simulink model "pmsm_model_Lab4_sensorless_st_R2022a"  (R2022a)
settings: Solver=ode4  StartTime=0.0  StopTime=Tf  FixedStep=Tsim  MaxStep=Tsim  MinStep=Tsim/100  RelTol=1e-3
values from neighbouring files (symbols this model uses):
  b = 0    [pmsm_param_Lab4_2024_st.m]
  C32 = [ 1       0 ... (first row only)    [pmsm_param_Lab1_2025.m]    (also in pmsm_param_Lab2_2025_st.m; pmsm_param_Lab3_st.m; pmsm_param_Lab4_2024_st.m)
  C32inv = 2/3*[1    -1/2        -1/2 ... (first row only)    [pmsm_param_Lab1_2025.m]    (also in pmsm_param_Lab2_2025_st.m; pmsm_param_Lab3_st.m; pmsm_param_Lab4_2024_st.m)
  C33 = C32*C32inv    [pmsm_param_Lab1_2025.m]    (also in pmsm_param_Lab2_2025_st.m; pmsm_param_Lab3_st.m; pmsm_param_Lab4_2024_st.m)
  Cb = 500e-6    (= 0.0005)    [pmsm_param_Lab3_st.m]    (also in pmsm_param_Lab4_2024_st.m)
  dTm0 = 0.20*Tmrated    (= 48)    [pmsm_param_Lab2_2025_st.m]    (also in pmsm_param_Lab3_st.m; pmsm_param_Lab4_2024_st.m = 120)
  Dyno = 1    [pmsm_param_Lab3_st.m]    (also in pmsm_param_Lab4_2024_st.m = 0)
  f = 15e-3    (= 0.015)    [pmsm_param_Lab1_2025.m]    (also in pmsm_param_Lab2_2025_st.m; pmsm_param_Lab3_st.m; pmsm_param_Lab4_2024_st.m)
  frslvr = 1/Ts    (= 10000)    [pmsm_param_Lab4_2024_st.m]
  Id0 = 0    [pmsm_param_Lab1_2025.m]    (also in pmsm_param_Lab2_2025_st.m; pmsm_param_Lab3_st.m = interp1(Tref,Idopt,Tm0); pmsm_param_Lab4_2024_st.m = interp1(Tref,Idopt,Tm0))
  Idc0 = Pe0/VDC    [pmsm_param_Lab3_st.m]    (also in pmsm_param_Lab4_2024_st.m)
  Idopt = zeros(1,NT)    [pmsm_param_Lab3_st.m]    (also in pmsm_param_Lab4_2024_st.m)
  Iq0 = 2/3*Tm0/(Pp*Psif)    (= 0)    [pmsm_param_Lab1_2025.m]    (also in pmsm_param_Lab2_2025_st.m = 119.926066866; pmsm_param_Lab3_st.m = interp1(Tref,Iqopt,Tm0); pmsm_param_Lab4_2024_st.m = interp1(Tref,Iqopt,Tm0))
  Iqopt = zeros(1,NT)    [pmsm_param_Lab3_st.m]    (also in pmsm_param_Lab4_2024_st.m)
  J = 100e-3    (= 0.1)    [pmsm_param_Lab1_2025.m]    (also in pmsm_param_Lab2_2025_st.m; pmsm_param_Lab3_st.m; pmsm_param_Lab4_2024_st.m)
  Kid = Kpd / tid    (= 282.743237724)    [pmsm_param_Lab2_2025_st.m]    (also in pmsm_param_Lab3_st.m = 180; pmsm_param_Lab4_2024_st.m = 180)
  Kiq = Kpq / tiq    (= 282.743237724)    [pmsm_param_Lab2_2025_st.m]    (also in pmsm_param_Lab3_st.m = 180; pmsm_param_Lab4_2024_st.m = 180)
  kL = 0.750    (= 0.75)    [pmsm_param_Lab1_2025.m]    (also in pmsm_param_Lab2_2025_st.m; pmsm_param_Lab3_st.m; pmsm_param_Lab4_2024_st.m)
  Kpd = (3*Ld0) / tr    (= 6.28318306054)    [pmsm_param_Lab2_2025_st.m]    (also in pmsm_param_Lab3_st.m = 3; pmsm_param_Lab4_2024_st.m = 3)
  Kpll = 1    [pmsm_param_Lab4_2024_st.m]
  Kpq = (3 * Lq0) / tr    (= 3.14159153027)    [pmsm_param_Lab2_2025_st.m]    (also in pmsm_param_Lab3_st.m = 6; pmsm_param_Lab4_2024_st.m = 6)
  ksi = 0    [pmsm_param_Lab4_2024_st.m]
  Lb = 20e-6    (= 2e-05)    [pmsm_param_Lab3_st.m]    (also in pmsm_param_Lab4_2024_st.m)
  Ld0 = 2.0*Ld    (= 0.002)    [pmsm_param_Lab2_2025_st.m]    (also in pmsm_param_Lab3_st.m = 0.001; pmsm_param_Lab4_2024_st.m = 0.001)
  Lq0 = 0.5*Lq    (= 0.001)    [pmsm_param_Lab2_2025_st.m]    (also in pmsm_param_Lab3_st.m = 0.002; pmsm_param_Lab4_2024_st.m = 0.002)
  Pe0 = 3/2*(Vd0*Id0+Vq0*Iq0)    [pmsm_param_Lab2_2025_st.m]    (also in pmsm_param_Lab3_st.m; pmsm_param_Lab4_2024_st.m)
  Pp = 4    [pmsm_param_Lab1_2025.m]    (also in pmsm_param_Lab2_2025_st.m; pmsm_param_Lab3_st.m; pmsm_param_Lab4_2024_st.m)
  ppll = cell2mat(ppll)    [pmsm_param_Lab4_2024_st.m]
  Psid0 = interpn(Idv,Iqv,Psidd,Id0,Iq0)    [pmsm_param_Lab1_2025.m]    (also in pmsm_param_Lab2_2025_st.m; pmsm_param_Lab3_st.m; pmsm_param_Lab4_2024_st.m)
  Psif0 = 1.0*Psif    (= 0.167)    [pmsm_param_Lab2_2025_st.m]    (also in pmsm_param_Lab3_st.m; pmsm_param_Lab4_2024_st.m)
  Psiq0 = interpn(Idv,Iqv,Psiqq,Id0,Iq0)    [pmsm_param_Lab1_2025.m]    (also in pmsm_param_Lab2_2025_st.m; pmsm_param_Lab3_st.m; pmsm_param_Lab4_2024_st.m)
  Qbat = 72*3600    (= 259200)    [pmsm_param_Lab3_st.m]    (also in pmsm_param_Lab4_2024_st.m)
  RateTm = 10000    [pmsm_param_Lab3_st.m]    (also in pmsm_param_Lab4_2024_st.m)
  rb = 80e-3    (= 0.08)    [pmsm_param_Lab3_st.m]    (also in pmsm_param_Lab4_2024_st.m)
  Rs = 60e-3    (= 0.06)    [pmsm_param_Lab1_2025.m]    (also in pmsm_param_Lab2_2025_st.m; pmsm_param_Lab3_st.m; pmsm_param_Lab4_2024_st.m)
  Rs0 = 1.5*Rs    (= 0.09)    [pmsm_param_Lab2_2025_st.m]    (also in pmsm_param_Lab3_st.m = 0.06; pmsm_param_Lab4_2024_st.m = 0.06)
  SOC0 = 0.50    (= 0.5)    [pmsm_param_Lab3_st.m]    (also in pmsm_param_Lab4_2024_st.m)
  Thetae0 = 0    [pmsm_param_Lab1_2025.m]    (also in pmsm_param_Lab2_2025_st.m; pmsm_param_Lab3_st.m; pmsm_param_Lab4_2024_st.m)
  Tm0 = (kL+f)*Wm0    (= 0)    [pmsm_param_Lab1_2025.m]    (also in pmsm_param_Lab2_2025_st.m = 120.165919; pmsm_param_Lab3_st.m = 192.2654704; pmsm_param_Lab4_2024_st.m)
  Tp = 100e-6    (= 0.0001)    [pmsm_param_Lab2_2025_st.m]    (also in pmsm_param_Lab3_st.m; pmsm_param_Lab4_2024_st.m)
  Tref = -Tmax:Tmax/100:Tmax    [pmsm_param_Lab3_st.m]    (also in pmsm_param_Lab4_2024_st.m)
  Ts = Tsim    [pmsm_param_Lab2_2025_st.m]    (also in pmsm_param_Lab3_st.m = 0.0001; pmsm_param_Lab4_2024_st.m = 0.0001)
  Tsim = 1e-6    (= 1e-06)    [pmsm_param_Lab1_2025.m]    (also in pmsm_param_Lab2_2025_st.m = min([Tp Ts])/100; pmsm_param_Lab3_st.m = min([Tp Ts])/100; pmsm_param_Lab4_2024_st.m = min([Tp Ts])/100)
  TSS = Tstep+0.050    (= 0.1)    [pmsm_param_Lab3_st.m]    (also in pmsm_param_Lab4_2024_st.m)
  Tstep = 0.10    (= 0.1)    [pmsm_param_Lab2_2025_st.m]    (also in pmsm_param_Lab3_st.m = 0.05; pmsm_param_Lab4_2024_st.m = 0.05)
  Ud0 = Rs*Id0    (= 0)    [pmsm_param_Lab2_2025_st.m]    (also in pmsm_param_Lab3_st.m; pmsm_param_Lab4_2024_st.m)
  Uq0 = Rs*Iq0    (= 7.19556401196)    [pmsm_param_Lab2_2025_st.m]    (also in pmsm_param_Lab3_st.m = 11.5129024191; pmsm_param_Lab4_2024_st.m = Rs*Iq0)
  Vd0 = Rs*Id0-Pp*Psiq0*Wm0    [pmsm_param_Lab1_2025.m]    (also in pmsm_param_Lab2_2025_st.m = Ud0-Pp*Psiq0*Wm0; pmsm_param_Lab3_st.m = Ud0-Pp*Psiq0*Wm0; pmsm_param_Lab4_2024_st.m = Ud0-Pp*Psiq0*Wm0)
  VDC = 800    [pmsm_param_Lab2_2025_st.m]    (also in pmsm_param_Lab3_st.m; pmsm_param_Lab4_2024_st.m)
  VDC0 = 0.8*VDC    (= 640)    [pmsm_param_Lab3_st.m]    (also in pmsm_param_Lab4_2024_st.m)
  Vp = VDC/2    (= 400)    [pmsm_param_Lab2_2025_st.m]    (also in pmsm_param_Lab3_st.m; pmsm_param_Lab4_2024_st.m)
  Vq0 = Rs*Iq0+Pp*Psid0*Wm0    [pmsm_param_Lab1_2025.m]    (also in pmsm_param_Lab2_2025_st.m = Uq0+Pp*Psid0*Wm0; pmsm_param_Lab3_st.m = Uq0+Pp*Psid0*Wm0; pmsm_param_Lab4_2024_st.m = Uq0+Pp*Psid0*Wm0)
  we0 = Pp*Wm0    (= 0)    [pmsm_param_Lab4_2024_st.m]
  Wm0 = 0    [pmsm_param_Lab1_2025.m]    (also in pmsm_param_Lab2_2025_st.m = 157.079632679; pmsm_param_Lab3_st.m = 251.327412287; pmsm_param_Lab4_2024_st.m)
  zpll = cell2mat(zpll)    [pmsm_param_Lab4_2024_st.m]
undefined symbols (not defined in the file or in its folder): DiscIntNeverNeededParam, Idd, Idrop, Iqq, Isw, kpll, Psidv, Psiqv, SwLoss, Vdrop
libraries: simulink x10
(part 2 of 2)

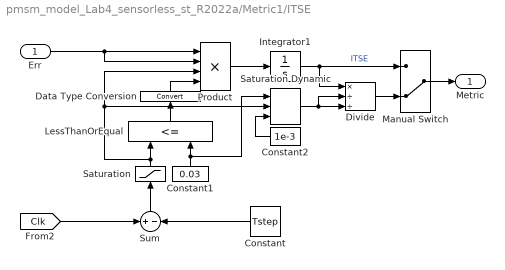
== system pmsm_model_Lab4_sensorless_st_R2022a/Metric1/ITSE ==
  Err : Inport
  Constant : Constant  Value=Tstep
  Constant1 : Constant  Value=0.03
  Constant2 : Constant  Value=1e-3
  Data Type Conversion : DataTypeConversion  SaturateOnIntegerOverflow=off  RndMeth=Floor
  Divide : Product  Inputs=*//
  Integrator1 : Integrator
  LessThanOrEqual : RelationalOperator  Operator=<=  OutDataTypeStr=boolean  RndMeth=Simplest  InputSameDT=off
  Manual Switch : ManualSwitch  CurrentSetting=0
  Product : Product  Inputs=4
  Saturation : Saturate  UpperLimit=inf  LowerLimit=0
  Saturation Dynamic : simulink/Discontinuities/Saturation Dynamic  OutMin=[]  OutMax=[]  OutDataTypeStr=Inherit: Same as second input  OutDataType=fixdt(1, 16)  OutScaling=2^-10  DoSatur=off
  Sum : Sum  Inputs=+|-
  Metric : Outport
  wires:
  Sum/1 -> Saturation/1
  Integrator1/1 -> Divide/1, Manual Switch/1  "ITSE"
  Err/1 -> Product/1, Product/2
  Product/1 -> Integrator1/1
  [Clk] -> Sum/1
  Saturation/1 -> Saturation Dynamic/2, Product/3, LessThanOrEqual/1
  Constant/1 -> Sum/2
  Divide/1 -> Manual Switch/2
  Manual Switch/1 -> Metric/1
  Saturation Dynamic/1 -> Divide/3, Divide/2
  LessThanOrEqual/1 -> Data Type Conversion/1
  Constant1/1 -> Saturation Dynamic/1, LessThanOrEqual/2
  Data Type Conversion/1 -> Product/4
  Constant2/1 -> Saturation Dynamic/3

== system pmsm_model_Lab4_sensorless_st_R2022a/Metric1/LPF ==
  x : Inport
  Gain : Gain  Gain=2*pi*10
  Integrator : Integrator
  Sum : Sum  Inputs=|+-
  xf : Outport
  wires:
  Gain/1 -> Integrator/1
  Sum/1 -> Gain/1
  Integrator/1 -> Sum/2, xf/1
  x/1 -> Sum/1

== system pmsm_model_Lab4_sensorless_st_R2022a/Metric1/RMSE ==
  Err : Inport
  Divide : Product  Inputs=*/
  Integrator1 : Integrator
  Integrator2 : Integrator
  Product : Product  Inputs=3
  Saturation : Saturate  UpperLimit=inf  LowerLimit=1e-3
  Sqrt : Sqrt
  Sqrt1 : Sqrt
  RMSE : Outport
  wires:
  Err/1 -> Product/1, Product/2
  Product/1 -> Integrator1/1
  Integrator1/1 -> Sqrt/1
  Sqrt/1 -> Divide/1
  [SS] -> Product/3, Integrator2/1
  Divide/1 -> RMSE/1
  Integrator2/1 -> Saturation/1
  Saturation/1 -> Sqrt1/1
  Sqrt1/1 -> Divide/2

== system pmsm_model_Lab4_sensorless_st_R2022a/Metric2/LPF ==
  Tm : Inport
  Gain : Gain  Gain=2*pi*10
  Integrator : Integrator  InitialCondition=Tm0
  Sum : Sum  Inputs=|+-
  Tav : Outport
  wires:
  Gain/1 -> Integrator/1
  Integrator/1 -> Tav/1, Sum/2
  Sum/1 -> Gain/1
  Tm/1 -> Sum/1

== system pmsm_model_Lab4_sensorless_st_R2022a/Metric2/Window ==
  "Tav " : Inport
  Dead Zone : DeadZone  LowerValue=-inf  UpperValue=Tstep
  Manual Switch : ManualSwitch
  Product : Product
  Tav : Outport
  wires:
  [SS] -> Manual Switch/1
  Dead Zone/1 -> Manual Switch/2  "ITSE"
  Manual Switch/1 -> Product/2
  Product/1 -> Tav/1
  [Clk] -> Dead Zone/1
  "Tav "/1 -> Product/1

== system pmsm_model_Lab4_sensorless_st_R2022a/Metric3/LPF ==
  Tm : Inport
  Gain : Gain  Gain=2*pi*30
  Integrator : Integrator  InitialCondition=Tm0
  Sum : Sum  Inputs=|+-
  Sum1 : Sum  Inputs=+-|
  Tmh : Outport
  Tm0 : Outport  Port=2
  wires:
  Tm/1 -> Sum1/1, Sum/1
  Integrator/1 -> Sum1/2, Tm0/1, Sum/2
  Sum/1 -> Gain/1
  Sum1/1 -> Tmh/1
  Gain/1 -> Integrator/1

== system pmsm_model_Lab4_sensorless_st_R2022a/Metric3/LPF2 ==
  x : Inport
  Gain : Gain  Gain=2*pi*10
  Integrator : Integrator
  Sum : Sum  Inputs=|+-
  xf : Outport
  wires:
  Gain/1 -> Integrator/1
  Sum/1 -> Gain/1
  Integrator/1 -> Sum/2, xf/1
  x/1 -> Sum/1

== system pmsm_model_Lab4_sensorless_st_R2022a/Metric3/Ripple ==
  Tmh : Inport
  Tm0 : Inport  Port=2
  Divide : Product  Inputs=*//
  Gain : Gain  Gain=100
  Integrator1 : Integrator
  Integrator2 : Integrator
  Product : Product  Inputs=3
  Saturation : Saturate  UpperLimit=inf  LowerLimit=1e-3
  Saturation1 : Saturate  UpperLimit=inf  LowerLimit=1e-3
  Sqrt : Sqrt
  Sqrt1 : Sqrt
  Ripple : Outport
  wires:
  Product/1 -> Integrator1/1
  Integrator1/1 -> Sqrt/1
  Sqrt/1 -> Divide/1
  [SS] -> Integrator2/1, Product/3
  Divide/1 -> Gain/1
  Gain/1 -> Ripple/1
  Integrator2/1 -> Saturation/1
  Saturation/1 -> Sqrt1/1
  Tm0/1 -> Saturation1/1
  Saturation1/1 -> Divide/3
  Sqrt1/1 -> Divide/2
  Tmh/1 -> Product/1, Product/2

== system pmsm_model_Lab4_sensorless_st_R2022a/PMSM/Flux_Current ==
  Psid : Inport
  Psiq : Inport  Port=2
  Id : Lookup_n-D  BreakpointsForDimension1=Psidv  BreakpointsForDimension2=Psiqv  Table=Idd  InternalRulePriority=Speed  RndMeth=Simplest
      settings: InputPortMap=u0,u1
  Iq : Lookup_n-D  BreakpointsForDimension1=Psidv  BreakpointsForDimension2=Psiqv  Table=Iqq  InternalRulePriority=Speed  RndMeth=Simplest
      settings: InputPortMap=u0,u1
  id : Outport
  iq : Outport  Port=2
  wires:
  Psiq/1 -> Iq/2, Id/2
  Psid/1 -> Iq/1, Id/1
  Iq/1 -> iq/1
  Id/1 -> id/1

== system pmsm_model_Lab4_sensorless_st_R2022a/PMSM/abc_dq ==
  abc : Inport
  sin_cos : Inport  Port=2
  Demux : Demux  Outputs=2
      settings: DisplayOption=none
  Demux1 : Demux  Outputs=2
      settings: DisplayOption=none
  Gain3 : Gain  Gain=C32inv  Multiplication=Matrix(K*u)  OutDataTypeStr=Inherit: Same as input  ParamDataTypeStr=Inherit: Same as input
  Mux : Mux  Inputs=2
  Product{,1..3} (4 alike) : Product  InputSameDT=on  RndMeth=Zero  SaturateOnIntegerOverflow=on  OutDataTypeStr=Inherit: Same as first input
  Sum : Sum  Inputs=|++  InputSameDT=on  SaturateOnIntegerOverflow=on  OutDataTypeStr=Inherit: Same as first input
  Sum1 : Sum  Inputs=|-+  InputSameDT=on  SaturateOnIntegerOverflow=on  OutDataTypeStr=Inherit: Same as first input
  dq : Outport
  wires:
  Sum1/1 -> Mux/2
  Mux/1 -> dq/1
  Demux1/1 -> Product2/2, Product1/2
  sin_cos/1 -> Demux1/1
  Demux/2 -> Product3/2, Product1/1
  Gain3/1 -> Demux/1  "alpha_beta"
  abc/1 -> Gain3/1
  Demux1/2 -> Product3/1, Product/2
  Demux/1 -> Product2/1, Product/1
  Sum/1 -> Mux/1
  Product3/1 -> Sum1/2
  Product2/1 -> Sum1/1
  Product1/1 -> Sum/2
  Product/1 -> Sum/1

== system pmsm_model_Lab4_sensorless_st_R2022a/PMSM/dq_abc ==
  dq : Inport
  sin_cos : Inport  Port=2
  Demux1 : Demux  Outputs=2
      settings: DisplayOption=none
  Demux2 : Demux  Outputs=2
      settings: DisplayOption=none
  Gain1 : Gain  Gain=C32  Multiplication=Matrix(K*u)  OutDataTypeStr=Inherit: Same as input  ParamDataTypeStr=Inherit: Same as input
  Mux : Mux  Inputs=2
  Product{,1..3} (4 alike) : Product  InputSameDT=on  RndMeth=Zero  SaturateOnIntegerOverflow=on  OutDataTypeStr=Inherit: Same as first input
  Sum : Sum  Inputs=|+-  InputSameDT=on  SaturateOnIntegerOverflow=on  OutDataTypeStr=Inherit: Same as first input
  Sum1 : Sum  Inputs=|++  InputSameDT=on  SaturateOnIntegerOverflow=on  OutDataTypeStr=Inherit: Same as first input
  abc : Outport
  wires:
  Mux/1 -> Gain1/1
  Demux1/1 -> Product2/2, Product1/2
  sin_cos/1 -> Demux1/1
  dq/1 -> Demux2/1
  Demux1/2 -> Product3/1, Product/2
  Product3/1 -> Sum1/2
  Product2/1 -> Sum1/1
  Product1/1 -> Sum/2
  Product/1 -> Sum/1
  Demux2/1 -> Product/1, Product2/1
  Demux2/2 -> Product3/2, Product1/1
  Sum/1 -> Mux/1
  Sum1/1 -> Mux/2
  Gain1/1 -> abc/1

== system pmsm_model_Lab4_sensorless_st_R2022a/PMSM/sin_cos ==
  thetae : Inport
  Mux1 : Mux  Inputs=2
  Trigonometric Function : Trigonometry
  Trigonometric Function1 : Trigonometry  Operator=cos
  sin_cos : Outport
  wires:
  Trigonometric Function/1 -> Mux1/1
  Trigonometric Function1/1 -> Mux1/2
  thetae/1 -> Trigonometric Function1/1, Trigonometric Function/1
  Mux1/1 -> sin_cos/1

== system pmsm_model_Lab4_sensorless_st_R2022a/Resolver/PLLPositionError ==
  u1 : Inport
  u2 : Inport  Port=2
  Constant : Constant  Value=2*pi
  Gain : Gain  Gain=0.5
  Sum : Sum  Inputs=+-+
  Sum1 : Sum  Inputs=-+|
  teta : Math  Operator=mod  SignedPower=on
  err : Outport
  wires:
  u2/1 -> Sum/2
  Sum/1 -> teta/1
  teta/1 -> Sum1/2
  Constant/1 -> Gain/1, teta/2
  Sum1/1 -> err/1
  u1/1 -> Sum/1
  Gain/1 -> Sum/3, Sum1/1

== system pmsm_model_Lab4_sensorless_st_R2022a/Resolver/PositionEstimationError ==
  u1 : Inport
  u2 : Inport  Port=2
  Constant : Constant  Value=2*pi
  Gain : Gain  Gain=0.5
  Sum : Sum  Inputs=+-+
  Sum1 : Sum  Inputs=-+|
  teta : Math  Operator=mod  SignedPower=on
  err : Outport
  wires:
  Gain/1 -> Sum1/1, Sum/3
  u1/1 -> Sum/1
  Sum1/1 -> err/1
  Constant/1 -> teta/2, Gain/1
  teta/1 -> Sum1/2
  Sum/1 -> teta/1
  u2/1 -> Sum/2

== system pmsm_model_Lab4_sensorless_st_R2022a/Resolver/SimplifiedResolver ==
  Thetae : Inport
  Supply : Inport  Port=2
  Product : Product
  Product1 : Product
  Sum : Sum  Inputs=++|
  Trigonometric Function : Trigonometry  Operator=cos
  Trigonometric Function1 : Trigonometry
  unbalalanced_gain : Gain
  unbalanced_offset : Constant  Value=0
  cosm : Outport
  sinm : Outport  Port=2
  wires:
  unbalalanced_gain/1 -> Sum/2
  Thetae/1 -> Trigonometric Function1/1, Trigonometric Function/1
  Trigonometric Function/1 -> unbalalanced_gain/1
  unbalanced_offset/1 -> Sum/1
  Trigonometric Function1/1 -> Product1/1
  Sum/1 -> Product/1
  Product/1 -> cosm/1
  Product1/1 -> sinm/1
  Supply/1 -> Product/2, Product1/2

== system pmsm_model_Lab4_sensorless_st_R2022a/SPWM/S1 ==
  "C " : Inport
  NOT : Logic  Operator=NOT  IconShape=distinctive  AllPortsSameDT=off  OutDataTypeStr=boolean
  C : Outport
  C* : Outport  Port=2
  wires:
  "C "/1 -> C/1, NOT/1
  NOT/1 -> C*/1

== system pmsm_model_Lab4_sensorless_st_R2022a/SPWM/S2 ==
  "C " : Inport
  NOT : Logic  Operator=NOT  IconShape=distinctive  AllPortsSameDT=off  OutDataTypeStr=boolean
  C : Outport
  C* : Outport  Port=2
  wires:
  NOT/1 -> C*/1
  "C "/1 -> NOT/1, C/1

== system pmsm_model_Lab4_sensorless_st_R2022a/SPWM/S3 ==
  "C " : Inport
  NOT : Logic  Operator=NOT  IconShape=distinctive  AllPortsSameDT=off  OutDataTypeStr=boolean
  C : Outport
  C* : Outport  Port=2
  wires:
  "C "/1 -> C/1, NOT/1
  NOT/1 -> C*/1

== system pmsm_model_Lab4_sensorless_st_R2022a/SPWM/carrier ==
  t : Inport
  Abs : Abs
  Constant2 : Constant  Value=-Vp
  Signal Generator : SignalGenerator  WaveForm=sawtooth  TimeSource=Use external signal  Amplitude=2*Vp  Frequency=1/Tp
  Sum2 : Sum  SaturateOnIntegerOverflow=on
  Vp : Outport
  wires:
  Sum2/1 -> Vp/1
  Constant2/1 -> Sum2/1
  Abs/1 -> Sum2/2
  Signal Generator/1 -> Abs/1
  t/1 -> Signal Generator/1

== system pmsm_model_Lab4_sensorless_st_R2022a/VSI/V1 ==
  C : Inport
  C* : Inport  Port=2
  I : Inport  Port=3
  Vs : Inport  Port=4
  Compare To Zero : simulink/Logic and Bit Operations/Compare To Zero  relop=>  OutDataTypeStr=boolean  ZeroCross=off
  Demux : Demux  Outputs=2
  Leg : CombinatorialLogic  TruthTable=[1 1;0 0;1 1;0.5 1;0 0;0 0;1 1;0.5 1]
  Mux : Mux  Inputs=3
  Product1 : Product  SaturateOnIntegerOverflow=on  OutDataTypeStr=Inherit: Same as first input
  Product3 : Product  SaturateOnIntegerOverflow=on  OutDataTypeStr=Inherit: Same as first input
  Sum1 : Sum  Inputs=-+|  SaturateOnIntegerOverflow=on
  Vdrop : Lookup_n-D  NumberOfTableDimensions=1  BreakpointsForDimension1=Idrop  Table=Vdrop  InternalRulePriority=Speed  RndMeth=Simplest
  V : Outport
  il : Outport  Port=2
  wires:
  Mux/1 -> Leg/1
  I/1 -> Product3/2, Vdrop/1, Compare To Zero/1
  C*/1 -> Mux/3
  C/1 -> Mux/2
  Compare To Zero/1 -> Mux/1
  Leg/1 -> Demux/1
  Demux/1 -> Product1/2
  Vs/1 -> Product1/1
  Sum1/1 -> V/1
  Product3/1 -> il/1
  Demux/2 -> Product3/1
  Product1/1 -> Sum1/2
  Vdrop/1 -> Sum1/1

== system pmsm_model_Lab4_sensorless_st_R2022a/VSI/V2 ==
  C : Inport
  C* : Inport  Port=2
  I : Inport  Port=3
  Vs : Inport  Port=4
  Compare To Zero : simulink/Logic and Bit Operations/Compare To Zero  relop=>  OutDataTypeStr=boolean  ZeroCross=off
  Demux : Demux  Outputs=2
  Leg : CombinatorialLogic  TruthTable=[1 1;0 0;1 1;0.5 1;0 0;0 0;1 1;0.5 1]
  Mux : Mux  Inputs=3
  Product1 : Product  SaturateOnIntegerOverflow=on  OutDataTypeStr=Inherit: Same as first input
  Product3 : Product  SaturateOnIntegerOverflow=on  OutDataTypeStr=Inherit: Same as first input
  Sum1 : Sum  Inputs=-+|  SaturateOnIntegerOverflow=on
  Vdrop : Lookup_n-D  NumberOfTableDimensions=1  BreakpointsForDimension1=Idrop  Table=Vdrop  InternalRulePriority=Speed  RndMeth=Simplest
  V : Outport
  il : Outport  Port=2
  wires:
  Vdrop/1 -> Sum1/1
  Product1/1 -> Sum1/2
  Demux/2 -> Product3/1
  Product3/1 -> il/1
  Sum1/1 -> V/1
  Vs/1 -> Product1/1
  Demux/1 -> Product1/2
  Leg/1 -> Demux/1
  Compare To Zero/1 -> Mux/1
  C/1 -> Mux/2
  C*/1 -> Mux/3
  I/1 -> Compare To Zero/1, Vdrop/1, Product3/2
  Mux/1 -> Leg/1

== system pmsm_model_Lab4_sensorless_st_R2022a/VSI/V3 ==
  C : Inport
  C* : Inport  Port=2
  I : Inport  Port=3
  Vs : Inport  Port=4
  Compare To Zero : simulink/Logic and Bit Operations/Compare To Zero  relop=>  OutDataTypeStr=boolean  ZeroCross=off
  Demux : Demux  Outputs=2
  Leg : CombinatorialLogic  TruthTable=[1 1;0 0;1 1;0.5 1;0 0;0 0;1 1;0.5 1]
  Mux : Mux  Inputs=3
  Product1 : Product  SaturateOnIntegerOverflow=on  OutDataTypeStr=Inherit: Same as first input
  Product3 : Product  SaturateOnIntegerOverflow=on  OutDataTypeStr=Inherit: Same as first input
  Sum1 : Sum  Inputs=-+|  SaturateOnIntegerOverflow=on
  Vdrop : Lookup_n-D  NumberOfTableDimensions=1  BreakpointsForDimension1=Idrop  Table=Vdrop  InternalRulePriority=Speed  RndMeth=Simplest
  V : Outport
  il : Outport  Port=2
  wires:
  Mux/1 -> Leg/1
  I/1 -> Product3/2, Vdrop/1, Compare To Zero/1
  C*/1 -> Mux/3
  C/1 -> Mux/2
  Compare To Zero/1 -> Mux/1
  Leg/1 -> Demux/1
  Demux/1 -> Product1/2
  Vs/1 -> Product1/1
  Sum1/1 -> V/1
  Product3/1 -> il/1
  Demux/2 -> Product3/1
  Product1/1 -> Sum1/2
  Vdrop/1 -> Sum1/1

== system pmsm_model_Lab4_sensorless_st_R2022a/VSI/VSI_Power ==
  V123 : Inport
  I1 : Inport  Port=2
  I2 : Inport  Port=3
  I3 : Inport  Port=4
  Iabc : Inport  Port=5
  Vdc : Inport  Port=6
  Idc : Scope
  Integrator : Integrator
  Product : Product
  Subsystem1 : Subsystem
  Sum : Sum  Inputs=+++
  Sum1 : Sum  Inputs=|++
  Sum2 : Sum  Inputs=|++
  Edc : Outport
  Pdc : Outport  Port=2
  wires:
  Product/1 -> Sum2/2, Integrator/1
  V123/1 -> Subsystem1/1(V123)
  Sum/1 -> Product/1, Idc/1
  I1/1 -> Sum/1
  Subsystem1/2(SwLossP) -> Sum2/1
  I2/1 -> Sum/2
  Integrator/1 -> Sum1/2
  I3/1 -> Sum/3
  Vdc/1 -> Product/2
  Sum1/1 -> Edc/1
  Sum2/1 -> Pdc/1
  Iabc/1 -> Subsystem1/2(Iabc)
  Subsystem1/1(SwLossE) -> Sum1/1

== system pmsm_model_Lab4_sensorless_st_R2022a/Control/DiscreteR//D/FaultGeneration ==
  F : Inport
  Clear : Inport  Port=2
  Data Type Conversion{,1..4} (5 alike) : DataTypeConversion  SaturateOnIntegerOverflow=off  RndMeth=Floor
  Delay : Delay  DelayLength=1
  Delay1 : Delay  DelayLength=1
  Delay2 : Delay  DelayLength=1
  Logical Operator : Logic  Inputs=3  AllPortsSameDT=off  OutDataTypeStr=boolean
  Logical Operator1 : Logic  Operator=OR  AllPortsSameDT=off  OutDataTypeStr=boolean
  Logical Operator2 : Logic  AllPortsSameDT=off  OutDataTypeStr=boolean
  Logical Operator3 : Logic  Operator=NOT  AllPortsSameDT=off  OutDataTypeStr=boolean
  Fault : Outport
  wires:
  Delay2/1 -> Logical Operator1/2
  Data Type Conversion1/1 -> Logical Operator/2
  Delay/1 -> Delay1/1, Data Type Conversion1/1
  F/1 -> Delay/1, Data Type Conversion2/1
  Data Type Conversion/1 -> Logical Operator/3
  Logical Operator2/1 -> Delay2/1, Data Type Conversion3/1
  Data Type Conversion2/1 -> Logical Operator/1
  Logical Operator/1 -> Logical Operator1/1
  Logical Operator1/1 -> Logical Operator2/1
  Delay1/1 -> Data Type Conversion/1
  Data Type Conversion3/1 -> Fault/1
  Clear/1 -> Data Type Conversion4/1
  Data Type Conversion4/1 -> Logical Operator3/1
  Logical Operator3/1 -> Logical Operator2/2

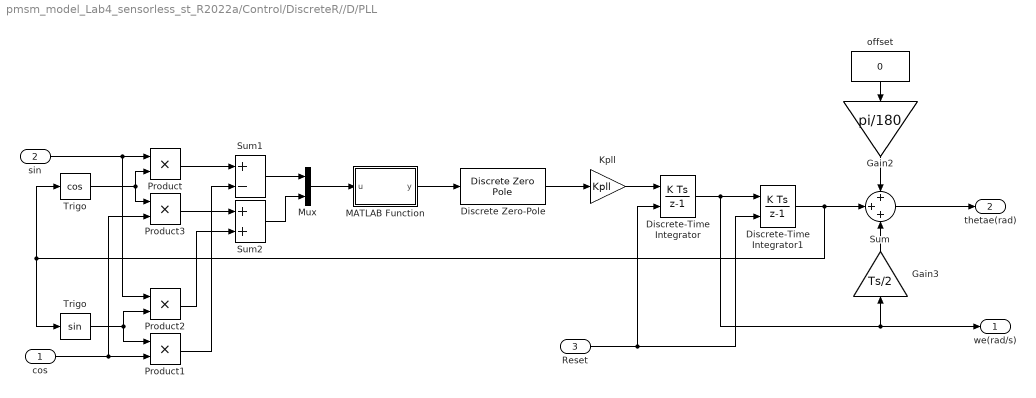
== system pmsm_model_Lab4_sensorless_st_R2022a/Control/DiscreteR//D/PLL ==
  cos : Inport
  sin : Inport  Port=2
  Reset : Inport  Port=3
  Discrete Zero-Pole : DiscreteZeroPole  Zeros=zpll  Poles=ppll  Gain=kpll  SampleTime=-1
  Discrete-Time Integrator : DiscreteIntegrator  ExternalReset=level  InitialCondition=Pp*Wm0  SampleTime=-1  ICPrevOutput=DiscIntNeverNeededParam  ICPrevScaledInput=DiscIntNeverNeededParam
  Discrete-Time Integrator1 : DiscreteIntegrator  ExternalReset=level  InitialCondition=Thetae0  SampleTime=-1  ICPrevOutput=DiscIntNeverNeededParam  ICPrevScaledInput=DiscIntNeverNeededParam
  Gain2 : Gain  Gain=pi/180  SaturateOnIntegerOverflow=on  OutDataTypeStr=Inherit: Same as input  ParamDataTypeStr=Inherit: Same as input
  Gain3 : Gain  Gain=Ts/2
  Kpll : Gain  Gain=Kpll
  MATLAB Function : MATLAB Function  TreatAsAtomicUnit=on
  Mux : Mux  Inputs=2
  Product{,1..3} (4 alike) : Product  SaturateOnIntegerOverflow=on  OutDataTypeStr=Inherit: Same as first input
  Sum : Sum  Inputs=+++  OutDataTypeStr=double  SaturateOnIntegerOverflow=on
  Sum1 : Sum  Inputs=+-  SaturateOnIntegerOverflow=on
  Sum2 : Sum  SaturateOnIntegerOverflow=on
  Trigo : Trigonometry  Operator=cos
  "Trigo " : Trigonometry
  offset : Constant  Value=0
  we(rad/s) : Outport
  thetae(rad) : Outport  Port=2
  wires:
  sin/1 -> Product2/1, Product/1
  cos/1 -> Product3/2, Product1/2
  Product/1 -> Sum1/1
  "Trigo "/1 -> Product2/2, Product1/1
  Trigo/1 -> Product3/1, Product/2
  Sum1/1 -> Mux/1
  offset/1 -> Gain2/1
  Gain2/1 -> Sum/1
  Sum/1 -> thetae(rad)/1
  Reset/1 -> Discrete-Time Integrator1/2, Discrete-Time Integrator/2
  Discrete-Time Integrator/1 -> Discrete-Time Integrator1/1, we(rad/s)/1, Gain3/1
  Discrete Zero-Pole/1 -> Kpll/1
  Kpll/1 -> Discrete-Time Integrator/1
  Gain3/1 -> Sum/3
  Discrete-Time Integrator1/1 -> Trigo/1, "Trigo "/1, Sum/2
  Product3/1 -> Sum2/1
  Mux/1 -> MATLAB Function/1(u)
  Sum2/1 -> Mux/2
  MATLAB Function/1(y) -> Discrete Zero-Pole/1
  Product1/1 -> Sum1/2
  Product2/1 -> Sum2/2

== system pmsm_model_Lab4_sensorless_st_R2022a/Control/dq to abc1/THIPWM ==
  Vabc* : Inport
  Add : Sum
  Add1 : Sum  Inputs=-+
  Gain : Gain  Gain=0.5
  MinMax1 : MinMax  InputSameDT=on  SaturateOnIntegerOverflow=on
  MinMax2 : MinMax  Function=max  InputSameDT=on  SaturateOnIntegerOverflow=on
  Vabc3* : Outport
  wires:
  Vabc*/1 -> MinMax1/1, Add1/2, MinMax2/1
  MinMax2/1 -> Add/2
  Add/1 -> Gain/1
  Gain/1 -> Add1/1
  Add1/1 -> Vabc3*/1
  MinMax1/1 -> Add/1

== system pmsm_model_Lab4_sensorless_st_R2022a/Control/sensorless/abc to dq1 ==
  "albt " : Inport
  sin_cos : Inport  Port=2
  Demux : Demux  Outputs=2
      settings: DisplayOption=none
  Demux1 : Demux  Outputs=2
      settings: DisplayOption=none
  Mux : Mux  Inputs=2
  Product{,1..3} (4 alike) : Product  InputSameDT=on  RndMeth=Zero  SaturateOnIntegerOverflow=on  OutDataTypeStr=Inherit: Same as first input
  Sum : Sum  Inputs=|++  InputSameDT=on  SaturateOnIntegerOverflow=on  OutDataTypeStr=Inherit: Same as first input
  Sum1 : Sum  Inputs=|-+  InputSameDT=on  SaturateOnIntegerOverflow=on  OutDataTypeStr=Inherit: Same as first input
  dq : Outport
  wires:
  Product/1 -> Sum/1
  Product1/1 -> Sum/2
  Product2/1 -> Sum1/1
  Product3/1 -> Sum1/2
  Sum/1 -> Mux/1
  Demux/1 -> Product/1, Product2/1
  Demux1/2 -> Product/2, Product3/1
  "albt "/1 -> Demux/1  "alpha_beta"
  Demux/2 -> Product1/1, Product3/2
  sin_cos/1 -> Demux1/1
  Demux1/1 -> Product1/2, Product2/2
  Mux/1 -> dq/1
  Sum1/1 -> Mux/2

== system pmsm_model_Lab4_sensorless_st_R2022a/Control/sensorless/abc to dq2 ==
  "albt " : Inport
  sin_cos : Inport  Port=2
  Demux : Demux  Outputs=2
      settings: DisplayOption=none
  Demux1 : Demux  Outputs=2
      settings: DisplayOption=none
  Mux : Mux  Inputs=2
  Product{,1..3} (4 alike) : Product  InputSameDT=on  RndMeth=Zero  SaturateOnIntegerOverflow=on  OutDataTypeStr=Inherit: Same as first input
  Sum : Sum  Inputs=|++  InputSameDT=on  SaturateOnIntegerOverflow=on  OutDataTypeStr=Inherit: Same as first input
  Sum1 : Sum  Inputs=|-+  InputSameDT=on  SaturateOnIntegerOverflow=on  OutDataTypeStr=Inherit: Same as first input
  dq : Outport
  wires:
  Product/1 -> Sum/1
  Product1/1 -> Sum/2
  Product2/1 -> Sum1/1
  Product3/1 -> Sum1/2
  Sum/1 -> Mux/1
  Demux/1 -> Product/1, Product2/1
  Demux1/2 -> Product/2, Product3/1
  "albt "/1 -> Demux/1  "alpha_beta"
  Demux/2 -> Product1/1, Product3/2
  sin_cos/1 -> Demux1/1
  Demux1/1 -> Product1/2, Product2/2
  Mux/1 -> dq/1
  Sum1/1 -> Mux/2

== system pmsm_model_Lab4_sensorless_st_R2022a/Control/sensorless/sin_cos ==
  thetae : Inport
  Mux1 : Mux  Inputs=2
  Trigonometric Function : Trigonometry
  Trigonometric Function1 : Trigonometry  Operator=cos
  sin_cos : Outport
  wires:
  Trigonometric Function/1 -> Mux1/1
  Trigonometric Function1/1 -> Mux1/2
  thetae/1 -> Trigonometric Function1/1, Trigonometric Function/1
  Mux1/1 -> sin_cos/1

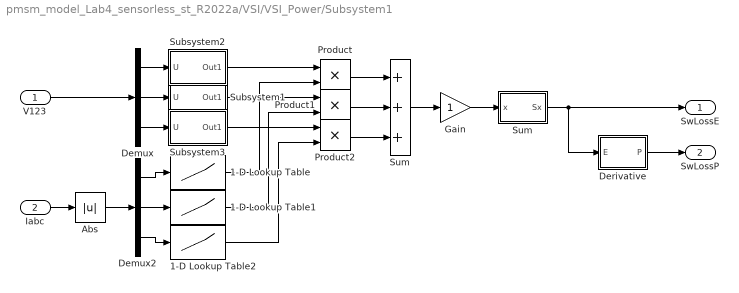
== system pmsm_model_Lab4_sensorless_st_R2022a/VSI/VSI_Power/Subsystem1 ==
  V123 : Inport
  Iabc : Inport  Port=2
  1-D Lookup Table : Lookup_n-D  NumberOfTableDimensions=1  BreakpointsForDimension1=Isw  Table=SwLoss  InternalRulePriority=Speed  RndMeth=Simplest
  1-D Lookup Table1 : Lookup_n-D  NumberOfTableDimensions=1  BreakpointsForDimension1=Isw  Table=SwLoss  InternalRulePriority=Speed  RndMeth=Simplest
  1-D Lookup Table2 : Lookup_n-D  NumberOfTableDimensions=1  BreakpointsForDimension1=Isw  Table=SwLoss  InternalRulePriority=Speed  RndMeth=Simplest
  Abs : Abs  SaturateOnIntegerOverflow=off
  Demux : Demux  Outputs=3
  Demux2 : Demux  Outputs=3
  Derivative : Subsystem
  Gain : Gain
  Product : Product
  Product1 : Product
  Product2 : Product
  Subsystem1 : Subsystem
  Subsystem2 : Subsystem
  Subsystem3 : Subsystem
  Sum : Sum  Inputs=+++
  "Sum " : Subsystem
  SwLossE : Outport
  SwLossP : Outport  Port=2
  wires:
  V123/1 -> Demux/1
  Abs/1 -> Demux2/1
  Demux2/3 -> 1-D Lookup Table2/1
  Demux2/2 -> 1-D Lookup Table1/1
  Demux2/1 -> 1-D Lookup Table/1
  Product2/1 -> Sum/3
  Product1/1 -> Sum/2
  Product/1 -> Sum/1
  Subsystem1/1(Out1) -> Product1/1
  Subsystem3/1(Out1) -> Product2/1
  Iabc/1 -> Abs/1
  Sum/1 -> Gain/1
  Subsystem2/1(Out1) -> Product/1
  Demux/3 -> Subsystem3/1(U)
  Demux/2 -> Subsystem1/1(U)
  Demux/1 -> Subsystem2/1(U)
  1-D Lookup Table/1 -> Product/2
  1-D Lookup Table1/1 -> Product1/2
  1-D Lookup Table2/1 -> Product2/2
  Derivative/1(P) -> SwLossP/1
  "Sum "/1(Sx) -> Derivative/1(E), SwLossE/1
  Gain/1 -> "Sum "/1(x)

== system pmsm_model_Lab4_sensorless_st_R2022a/VSI/VSI_Power/Subsystem1/Derivative ==
  E : Inport
  Divide1 : Product  Inputs=/*
  Saturation : Saturate  UpperLimit=inf  LowerLimit=1e-9
  Sum2 : Sum  Inputs=|+-
  Sum5 : Sum  Inputs=+-|
  Unit Delay1 : UnitDelay  SampleTime=-1  HasFrameUpgradeWarning=on
  Unit Delay2 : UnitDelay  SampleTime=-1  HasFrameUpgradeWarning=on
  P : Outport
  wires:
  Unit Delay2/1 -> Sum5/2
  Saturation/1 -> Divide1/1
  [Clk] -> Sum5/1, Unit Delay2/1
  E/1 -> Unit Delay1/1, Sum2/1
  Unit Delay1/1 -> Sum2/2
  Sum5/1 -> Saturation/1
  Sum2/1 -> Divide1/2
  Divide1/1 -> P/1

== system pmsm_model_Lab4_sensorless_st_R2022a/VSI/VSI_Power/Subsystem1/Subsystem1 ==
  U : Inport
  Gain : Gain
  Gain1 : Gain
  Subsystem : Subsystem
  Subsystem1 : Subsystem
  Sum3 : Sum  Inputs=|++  SaturateOnIntegerOverflow=on
  Out1 : Outport
  wires:
  U/1 -> Subsystem/1(U), Subsystem1/1(U)
  Subsystem1/1(Out1) -> Gain1/1
  Subsystem/1(Out1) -> Gain/1
  Gain/1 -> Sum3/2
  Sum3/1 -> Out1/1
  Gain1/1 -> Sum3/1

== system pmsm_model_Lab4_sensorless_st_R2022a/VSI/VSI_Power/Subsystem1/Subsystem2 ==
  U : Inport
  Gain : Gain
  Gain1 : Gain
  Subsystem : Subsystem
  Subsystem1 : Subsystem
  Sum3 : Sum  Inputs=|++  SaturateOnIntegerOverflow=on
  Out1 : Outport
  wires:
  Gain1/1 -> Sum3/1
  Sum3/1 -> Out1/1
  Gain/1 -> Sum3/2
  Subsystem/1(Out1) -> Gain/1
  Subsystem1/1(Out1) -> Gain1/1
  U/1 -> Subsystem1/1(U), Subsystem/1(U)

== system pmsm_model_Lab4_sensorless_st_R2022a/VSI/VSI_Power/Subsystem1/Subsystem3 ==
  U : Inport
  Gain : Gain
  Gain1 : Gain
  Subsystem : Subsystem
  Subsystem1 : Subsystem
  Sum3 : Sum  Inputs=|++  SaturateOnIntegerOverflow=on
  Out1 : Outport
  wires:
  Gain1/1 -> Sum3/1
  Sum3/1 -> Out1/1
  Gain/1 -> Sum3/2
  Subsystem/1(Out1) -> Gain/1
  Subsystem1/1(Out1) -> Gain1/1
  U/1 -> Subsystem1/1(U), Subsystem/1(U)

== system pmsm_model_Lab4_sensorless_st_R2022a/VSI/VSI_Power/Subsystem1/Sum  ==
  x : Inport
  Memory : Memory
  Sum1 : Sum  Inputs=|++
  Sx : Outport
  wires:
  Memory/1 -> Sum1/2
  x/1 -> Sum1/1
  Sum1/1 -> Memory/1, Sx/1

== system pmsm_model_Lab4_sensorless_st_R2022a/VSI/VSI_Power/Subsystem1/Subsystem1/Subsystem ==
  U : Inport
  Compare To Constant : simulink/Logic and Bit Operations/Compare To Constant  relop=<  const=-VDC0  OutDataTypeStr=uint8
  Memory : Memory
  Sum : Sum  Inputs=+-|
  Out1 : Outport
  wires:
  Compare To Constant/1 -> Out1/1
  U/1 -> Sum/1, Memory/1
  Sum/1 -> Compare To Constant/1
  Memory/1 -> Sum/2

== system pmsm_model_Lab4_sensorless_st_R2022a/VSI/VSI_Power/Subsystem1/Subsystem1/Subsystem1 ==
  U : Inport
  Compare To Constant : simulink/Logic and Bit Operations/Compare To Constant  relop=>  const=VDC0  OutDataTypeStr=uint8
  Memory : Memory
  Sum : Sum  Inputs=+-|
  Out1 : Outport
  wires:
  Compare To Constant/1 -> Out1/1
  Memory/1 -> Sum/2
  Sum/1 -> Compare To Constant/1
  U/1 -> Sum/1, Memory/1

== system pmsm_model_Lab4_sensorless_st_R2022a/VSI/VSI_Power/Subsystem1/Subsystem2/Subsystem ==
  U : Inport
  Compare To Constant : simulink/Logic and Bit Operations/Compare To Constant  relop=<  const=-VDC0  OutDataTypeStr=uint8
  Memory : Memory
  Sum : Sum  Inputs=+-|
  Out1 : Outport
  wires:
  Memory/1 -> Sum/2
  Sum/1 -> Compare To Constant/1
  U/1 -> Memory/1, Sum/1
  Compare To Constant/1 -> Out1/1

== system pmsm_model_Lab4_sensorless_st_R2022a/VSI/VSI_Power/Subsystem1/Subsystem2/Subsystem1 ==
  U : Inport
  Compare To Constant : simulink/Logic and Bit Operations/Compare To Constant  relop=>  const=VDC0  OutDataTypeStr=uint8
  Memory : Memory
  Sum : Sum  Inputs=+-|
  Out1 : Outport
  wires:
  U/1 -> Memory/1, Sum/1
  Sum/1 -> Compare To Constant/1
  Memory/1 -> Sum/2
  Compare To Constant/1 -> Out1/1

== system pmsm_model_Lab4_sensorless_st_R2022a/VSI/VSI_Power/Subsystem1/Subsystem3/Subsystem ==
  U : Inport
  Compare To Constant : simulink/Logic and Bit Operations/Compare To Constant  relop=<  const=-VDC0  OutDataTypeStr=uint8
  Memory : Memory
  Sum : Sum  Inputs=+-|
  Out1 : Outport
  wires:
  Memory/1 -> Sum/2
  Sum/1 -> Compare To Constant/1
  U/1 -> Memory/1, Sum/1
  Compare To Constant/1 -> Out1/1

== system pmsm_model_Lab4_sensorless_st_R2022a/VSI/VSI_Power/Subsystem1/Subsystem3/Subsystem1 ==
  U : Inport
  Compare To Constant : simulink/Logic and Bit Operations/Compare To Constant  relop=>  const=VDC0  OutDataTypeStr=uint8
  Memory : Memory
  Sum : Sum  Inputs=+-|
  Out1 : Outport
  wires:
  U/1 -> Memory/1, Sum/1
  Sum/1 -> Compare To Constant/1
  Memory/1 -> Sum/2
  Compare To Constant/1 -> Out1/1

== matlab function pmsm_model_Lab4_sensorless_st_R2022a/Control/DiscreteR//D/PLL/MATLAB Function ==
  data: u input; y output
function y = fcn(u)

y=atan2(u(1),u(2));  % 2pi-arctangent PLL

== matlab function pmsm_model_Lab4_sensorless_st_R2022a/Control/Ctrl ==
  data: idref input; idm input; iqref input; iqm input; we input; Pp parameter; Psif0 parameter; Ld0 parameter; Lq0 parameter; Rs0 parameter; Ts parameter; vd output; vq output; Kpd parameter; Kpq parameter; Kid parameter; Kiq parameter; Id0 parameter; Iq0 parameter; Ud0 parameter; Uq0 parameter; Tm0 parameter; Vd0 parameter; Vq0 parameter
function [vd, vq]  = Ctrl(idref, idm, iqref, iqm, we, Pp, Psif0, Ld0, Lq0, Rs0, Ts, Kpd, Kpq, Kid, Kiq, Id0, Iq0, Ud0, Uq0, Tm0, Vd0, Vq0)

persistent interrd interrq 

if isempty(interrd), interrd = Ud0; end
if isempty(interrq), interrq = Uq0; end

errd=idref-idm;
errq=iqref-iqm;
interrd=interrd+Kid*errd*Ts;
interrq=interrq+Kiq*errq*Ts;
vd=Kpd*errd+interrd-Lq0*iqm*we;
vq=Kpq*errq+interrq+(Psif0+Ld0*idm)*we;

end

== matlab function pmsm_model_Lab4_sensorless_st_R2022a/Control/sensorless/MATLAB Function ==
  data: v input size=2; i input size=2; w input size=1; e output size=2; Rs0 parameter; Ld0 parameter; Lq0 parameter; Psif0 parameter; Thetae0 parameter; we0 parameter
function e = fcn(v, i, w, Rs0, Ld0, Lq0, Psif0, Thetae0, we0)

persistent edf egf 

if isempty(edf), edf=0; end
if isempty(egf), egf=0; end

ed=0;
eg=0;

adf=0.95;
agf=0.98;
edf=adf*edf+(1-adf)*ed;
egf=agf*egf+(1-agf)*eg;

e=[edf; egf];

== matlab function pmsm_model_Lab4_sensorless_st_R2022a/Control/sensorless/MATLAB Function1 ==
  data: e input; ws output; b parameter; Psif0 parameter; ksi parameter
function ws = fcn(e, b, Psif0, ksi)

ed=e(1);
eg=e(2);

ws=0;

== matlab function pmsm_model_Lab4_sensorless_st_R2022a/PMSM/dq-PMSM ==
  data: vd input; dPsid output; vq input; id input; iq input; Psid input; Psiq input; Omega input; TL input; dPsiq output; dOmega output; dTheta output; Rs input; Pp parameter; f parameter; J parameter; Tm output
function [dPsid, dPsiq, dOmega, dTheta, Tm] = PMSM(vd, vq, id, iq, Psid, Psiq, Omega, TL, Rs, Pp, f, J)

w=Pp*Omega;
Tm=(3/2)*Pp*(Psid*iq-Psiq*id);   % Clarke
% Tm=p*(Psid*iq-Psiq*id);       % Concordia

dPsid=vd-Rs*id+w*Psiq;
dPsiq=vq-Rs*iq-w*Psid;
dOmega=(Tm-f*Omega-TL)/J;
dTheta=w;

== matlab function pmsm_model_Lab4_sensorless_st_R2022a/Control/DiscreteR//D/MATLAB Function ==
  settings: updateMethod=DISCRETE
  data: c input; s input; F output; w input
function F = fcn(c, s, w)

F=0;
